simulink model "One_Shot_Simulation"  (R2018b)
settings: Solver=VariableStepAuto  StartTime=0.0  StopTime=3  RelTol=1e-3
undefined symbols (not defined in the file or in its folder): DiscIntNeverNeededParam
libraries: simulink x2, dspmtrx3 x1, truetime x1
settings Model: Creator=ortegafausto  LastModifiedBy=of
settings SFSimCC: SimUseLocalCustomCode=off
settings RTWCC: RTWUseLocalCustomCode=off
settings CodeAppCC: StateflowObjectComments=on
settings SimscapeCC: SimscapeNormalizeSystem=off

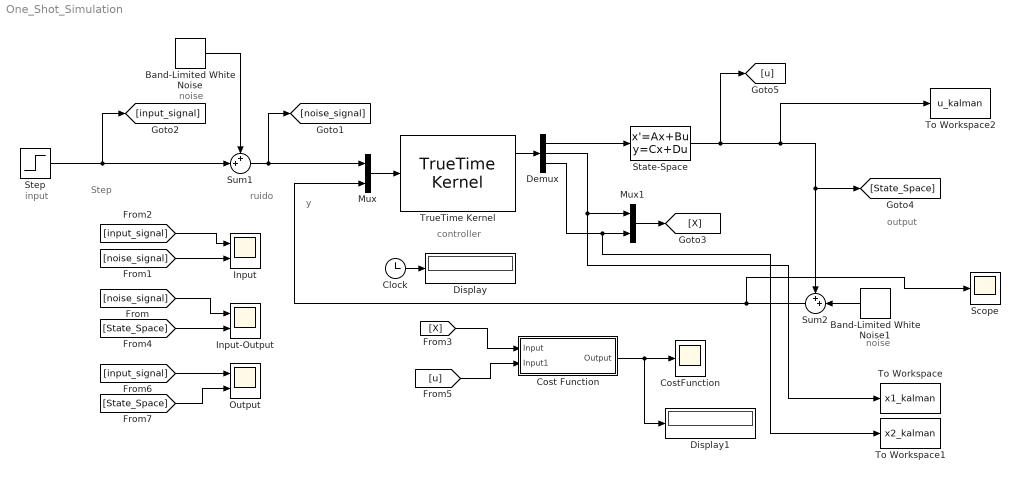
== system One_Shot_Simulation ==
  note: controller
  note: noise
  note: noise
  note: input
  note: output
  note: Step
  note: ruido
  note: y
  Band-Limited White Noise : simulink/Sources/Band-Limited White Noise  Cov=[0.0000005]  Ts=0.001  seed=[23341]
  Band-Limited White Noise1 : simulink/Sources/Band-Limited White Noise  Cov=[0.0000005]  Ts=0.001  seed=[23341]
  Clock : Clock
  Cost Function : Subsystem
  CostFunction : Scope
  Demux : Demux  Outputs=3
  Display : Display
  Display1 : Display
  "Input " : Scope  NumInputPorts=2
  "Input-Output " : Scope  NumInputPorts=2
  Mux : Mux  Inputs=2
  Mux1 : Mux  Inputs=2
  "Output " : Scope  NumInputPorts=2
  Scope : Scope
  State-Space : StateSpace  A=[0 1;-918 -90.9]  B=[0; 918.27]  C=[1 0]  D=0  InitialCondition=0
  Step : Step  Time=0.5  After=2.4  SampleTime=0
  Sum1 : Sum  Inputs=++|
  Sum2 : Sum  Inputs=++|
  To Workspace : ToWorkspace  VariableName=x1_kalman  SampleTime=-1
  To Workspace1 : ToWorkspace  VariableName=x2_kalman  SampleTime=-1
  To Workspace2 : ToWorkspace  VariableName=u_kalman  SampleTime=-1
  TrueTime Kernel : truetime/TrueTime Kernel  sfun=one_shot_init  args=[]  ninputsoutputs=[2 3]  ntriggers=0  trigtype=falling  nwnodenbr=[]  clockoffsetdrift=[0 0]  schedoutput=on  battery=off  poweroutput=off
  wires:
  Clock/1 -> Display/1
  Mux/1 -> TrueTime Kernel/1
  Step/1 -> Sum1/2, [input_signal]
  [noise_signal] -> "Input "/2
  [input_signal] -> "Input "/1
  [State_Space] -> "Input-Output "/2
  [input_signal] -> "Output "/1
  [State_Space] -> "Output "/2
  [noise_signal] -> "Input-Output "/1
  TrueTime Kernel/1 -> Demux/1
  Demux/1 -> State-Space/1
  Demux/2 -> To Workspace/1, Mux1/1
  Mux1/1 -> [X]
  [X] -> Cost Function/1(Input)
  [u] -> Cost Function/2(Input1)
  Cost Function/1(Output) -> Display1/1, CostFunction/1
  Sum1/1 -> Mux/1, [noise_signal]
  Band-Limited White Noise/1 -> Sum1/1
  State-Space/1 -> [u], To Workspace2/1, Sum2/1, [State_Space]
  Sum2/1 -> Scope/1, Mux/2
  Band-Limited White Noise1/1 -> Sum2/2
  Demux/3 -> To Workspace1/1, Mux1/2

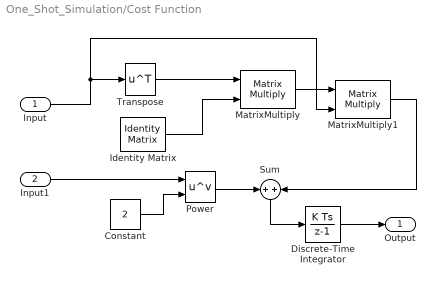
== system One_Shot_Simulation/Cost Function ==
  Input : Inport
  Input1 : Inport  Port=2
  Constant : Constant  Value=2
  Discrete-Time Integrator : DiscreteIntegrator  SampleTime=-1  ICPrevOutput=DiscIntNeverNeededParam  ICPrevScaledInput=DiscIntNeverNeededParam
  Identity Matrix : dspmtrx3/Identity Matrix  Inherit=off  N=2  Ts=1  dataType=double  isSigned=on  wordLen=16  udDataType=sfix(16)  fracBitsMode=Best precision  numFracBits=15  OutDataTypeStr=double  LastOutDataTypeStr=double
      settings: SourceProductName=DSP System Toolbox
  MatrixMultiply : Product  Multiplication=Matrix(*)
  MatrixMultiply1 : Product  Multiplication=Matrix(*)
  Power : Math  Operator=pow  SaturateOnIntegerOverflow=on
  Sum : Sum  Inputs=+|+
  Transpose : Math  Operator=transpose  SaturateOnIntegerOverflow=on
  Output : Outport
  wires:
  Identity Matrix/1 -> MatrixMultiply/2
  MatrixMultiply1/1 -> Sum/2
  Transpose/1 -> MatrixMultiply/1
  Power/1 -> Sum/1
  MatrixMultiply/1 -> MatrixMultiply1/1
  Discrete-Time Integrator/1 -> Output/1
  Sum/1 -> Discrete-Time Integrator/1
  Input/1 -> MatrixMultiply1/2, Transpose/1
  Input1/1 -> Power/1
  Constant/1 -> Power/2
